simulink model "CyclingProcess_v2"  (R2022a)
settings: Solver=VariableStepAuto  StartTime=0.0  StopTime=10.0  RelTol=1e-3
settings Model: Creator=mateu  LastModifiedBy=mateu

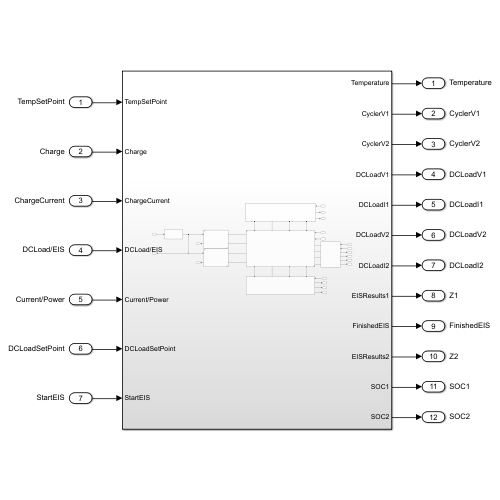
[thumbnail: Simulink's stored preview of the top-level diagram]
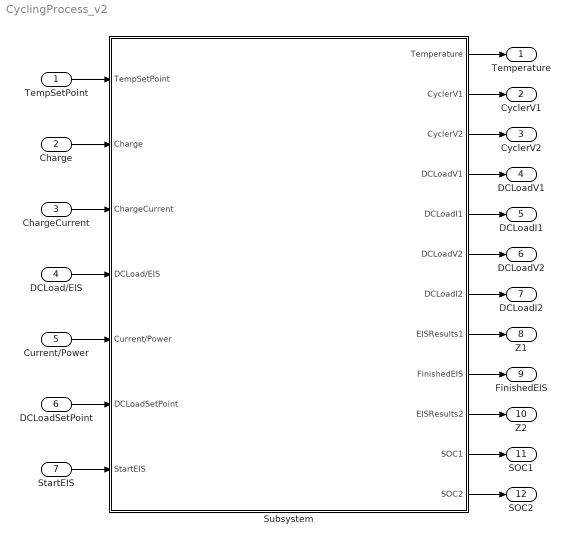
== system CyclingProcess_v2 ==
  TempSetPoint : Inport
  Charge : Inport  Port=2
  ChargeCurrent : Inport  Port=3
  DCLoad/EIS : Inport  Port=4
  Current/Power : Inport  Port=5
  DCLoadSetPoint : Inport  Port=6
  StartEIS : Inport  Port=7
  Subsystem : Subsystem
  Temperature : Outport
  CyclerV1 : Outport  Port=2
  CyclerV2 : Outport  Port=3
  DCLoadV1 : Outport  Port=4
  DCLoadI1 : Outport  Port=5
  DCLoadV2 : Outport  Port=6
  DCLoadI2 : Outport  Port=7
  Z1 : Outport  Port=8
  FinishedEIS : Outport  Port=9
  Z2 : Outport  Port=10
  SOC1 : Outport  Port=11
  SOC2 : Outport  Port=12
  wires:
  Subsystem/4(DCLoadV1) -> DCLoadV1/1
  Subsystem/7(DCLoadI2) -> DCLoadI2/1
  Subsystem/10(EISResults2) -> Z2/1
  Subsystem/12(SOC2) -> SOC2/1
  Subsystem/5(DCLoadI1) -> DCLoadI1/1
  Subsystem/11(SOC1) -> SOC1/1
  ChargeCurrent/1 -> Subsystem/3(ChargeCurrent)
  DCLoadSetPoint/1 -> Subsystem/6(DCLoadSetPoint)
  Subsystem/8(EISResults1) -> Z1/1
  Subsystem/3(CyclerV2) -> CyclerV2/1
  Charge/1 -> Subsystem/2(Charge)
  Subsystem/6(DCLoadV2) -> DCLoadV2/1
  Subsystem/1(Temperature) -> Temperature/1
  DCLoad/EIS/1 -> Subsystem/4(DCLoad/EIS)
  Current/Power/1 -> Subsystem/5(Current/Power)
  StartEIS/1 -> Subsystem/7(StartEIS)
  Subsystem/2(CyclerV1) -> CyclerV1/1
  TempSetPoint/1 -> Subsystem/1(TempSetPoint)
  Subsystem/9(FinishedEIS) -> FinishedEIS/1

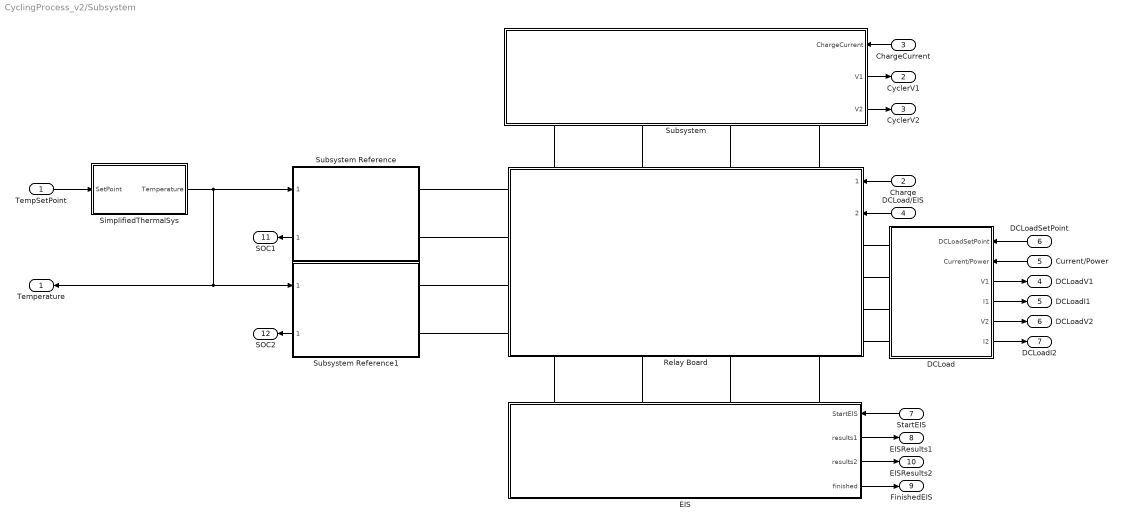
== system CyclingProcess_v2/Subsystem ==
  TempSetPoint : Inport
  Charge : Inport  Port=2
  ChargeCurrent : Inport  Port=3
  DCLoad/EIS : Inport  Port=4
  Current/Power : Inport  Port=5
  DCLoadSetPoint : Inport  Port=6
  StartEIS : Inport  Port=7
  DCLoad : Subsystem
      settings: PortSchema="{\"entries\":[{\"content\":{\"sides\":[{\"content\":{\"connectorIds\":[\"LConn1\",\"LConn2\",\"LConn3\",\"LConn4\"]},\"type\":\"ConnectorPlacement.EquallySpacedRectSide\",\"uuid\":\"7514b71b-63b4-4d0a-a4c6-1cc6fdc01e8b\"},{\"content\":{\"connectorIds\":[\"In1\",\"In2\",\"Out1\",\"Out2\",\"Out3\",\"Out4\"],\"side\":\"RIGHT\"},\"type\":\"ConnectorPlacement.EquallySpacedRectSide\",\"uuid\":\"8544a5e6-47c4-463c-a4b2-15ea7677f310\"},{\"content\":{\"connectorIds\":[],\"side\":\"TOP\"},\"type\":\"ConnectorPlacement.EquallySpacedRectSide\",\"uuid\":\"86aec749-4b5f-4df7-a96f-f425e3ea56a9\"}]},\"type\":\"ConnectorPlacement.EquallySpacedConnector\",\"uuid\":\"c9562699-1537-4762-a4d5-f653b7c21ddf\"}],\"packageUris\":[\"http://schema.mathworks.com/mf0/Connector/R2020b\"],\"version\":\"1.0\"}"
  EIS : Subsystem
      settings: PortSchema="{\"entries\":[{\"content\":{\"sides\":[{\"content\":{\"connectorIds\":[]},\"type\":\"ConnectorPlacement.EquallySpacedRectSide\",\"uuid\":\"cb9ec944-41ce-4636-a083-755c91ef9aeb\"},{\"content\":{\"connectorIds\":[\"In1\",\"Out1\",\"Out2\",\"Out3\"],\"side\":\"RIGHT\"},\"type\":\"ConnectorPlacement.EquallySpacedRectSide\",\"uuid\":\"d9055541-2ed5-47ee-9ebd-2502587374ee\"},{\"content\":{\"connectorIds\":[\"LConn1\",\"LConn2\",\"LConn3\",\"LConn4\"],\"side\":\"TOP\"},\"type\":\"ConnectorPlacement.EquallySpacedRectSide\",\"uuid\":\"957a55fb-9ef3-46c7-a91b-518a4a9602f1\"}]},\"type\":\"ConnectorPlacement.EquallySpacedConnector\",\"uuid\":\"9e8eff76-14a9-4e2b-897b-c7d74cf84e88\"}],\"packageUris\":[\"http://schema.mathworks.com/mf0/Connector/R2020b\"],\"version\":\"1.0\"}"
  Relay Board : Subsystem  ReferencedSubsystem=Relay_Board
      settings: PortSchema="{\"entries\":[{\"content\":{\"sides\":[{\"content\":{\"connectorIds\":[\"LConn1\",\"LConn2\",\"LConn3\",\"LConn4\"]},\"type\":\"ConnectorPlacement.EquallySpacedRectSide\",\"uuid\":\"b8d313c3-c08d-4f66-88c5-0966ca8ce19e\"},{\"content\":{\"connectorIds\":[\"In1\",\"In2\",\"RConn1\",\"RConn2\",\"RConn3\",\"RConn4\"],\"side\":\"RIGHT\"},\"type\":\"ConnectorPlacement.EquallySpacedRectSide\",\"uuid\":\"237515a3-1e1f-4c58-9863-54ac3610b1e3\"},{\"content\":{\"connectorIds\":[\"LConn5\",\"LConn6\",\"LConn7\",\"LConn8\"],\"side\":\"TOP\"},\"type\":\"ConnectorPlacement.EquallySpacedRectSide\",\"uuid\":\"521668e9-2c4f-424f-87c7-f56953ec1b76\"},{\"content\":{\"connectorIds\":[\"RConn5\",\"RConn6\",\"RConn7\",\"RConn8\"],\"side\":\"BOTTOM\"},\"type\":\"ConnectorPlacement.EquallySpacedRectSide\",\"uuid\":\"bf1ce9d0-6653-4dc3-bc27-a201294e6e6d\"}]},\"type\":\"ConnectorPlacement.EquallySpacedConnector\",\"uuid\":\"9b9e57dc-ee03-4c6e-905d-a66b18228b1b\"}],\"packageUris\":[\"http://schema.mathworks.com/mf0/Connector/R2020b\"],\"version\":\"1.0\"}"
  SimplifiedThermalSys : Subsystem
  Subsystem : Subsystem
      settings: PortSchema="{\"entries\":[{\"content\":{\"sides\":[{\"content\":{\"connectorIds\":[]},\"type\":\"ConnectorPlacement.EquallySpacedRectSide\",\"uuid\":\"cb9ec944-41ce-4636-a083-755c91ef9aeb\"},{\"content\":{\"connectorIds\":[\"In1\",\"Out1\",\"Out2\"],\"side\":\"RIGHT\"},\"type\":\"ConnectorPlacement.EquallySpacedRectSide\",\"uuid\":\"d9055541-2ed5-47ee-9ebd-2502587374ee\"},{\"content\":{\"connectorIds\":[],\"side\":\"TOP\"},\"type\":\"ConnectorPlacement.EquallySpacedRectSide\",\"uuid\":\"957a55fb-9ef3-46c7-a91b-518a4a9602f1\"},{\"content\":{\"connectorIds\":[\"RConn1\",\"RConn2\",\"RConn3\",\"RConn4\"],\"side\":\"BOTTOM\"},\"type\":\"ConnectorPlacement.EquallySpacedRectSide\",\"uuid\":\"144f5416-dcfd-4dc1-81f1-ec8b48bee9a2\"}]},\"type\":\"ConnectorPlacement.EquallySpacedConnector\",\"uuid\":\"9e8eff76-14a9-4e2b-897b-c7d74cf84e88\"}],\"packageUris\":[\"http://schema.mathworks.com/mf0/Connector/R2020b\"],\"version\":\"1.0\"}"
  Subsystem Reference : Subsystem  ReferencedSubsystem=Battery
      settings: PortSchema="{\"entries\":[{\"content\":{\"sides\":[{\"content\":{\"connectorIds\":[\"In1\",\"Out1\"]},\"type\":\"ConnectorPlacement.EquallySpacedRectSide\",\"uuid\":\"fc03161e-b2e2-4ac7-873d-06369879f611\"},{\"content\":{\"connectorIds\":[\"LConn1\",\"LConn2\"],\"side\":\"RIGHT\"},\"type\":\"ConnectorPlacement.EquallySpacedRectSide\",\"uuid\":\"979b6df9-5e16-4e4c-95de-06d721c40976\"},{\"content\":{\"connectorIds\":[],\"side\":\"TOP\"},\"type\":\"ConnectorPlacement.EquallySpacedRectSide\",\"uuid\":\"144c0b06-ab1a-42a6-a8bb-d1b96a840cfc\"}]},\"type\":\"ConnectorPlacement.EquallySpacedConnector\",\"uuid\":\"6783069b-24d2-410c-99c7-607924147892\"}],\"packageUris\":[\"http://schema.mathworks.com/mf0/Connector/R2020b\"],\"version\":\"1.0\"}"
  Subsystem Reference1 : Subsystem  ReferencedSubsystem=Battery
      settings: PortSchema="{\"entries\":[{\"content\":{\"sides\":[{\"content\":{\"connectorIds\":[\"In1\",\"Out1\"]},\"type\":\"ConnectorPlacement.EquallySpacedRectSide\",\"uuid\":\"fc03161e-b2e2-4ac7-873d-06369879f611\"},{\"content\":{\"connectorIds\":[\"LConn1\",\"LConn2\"],\"side\":\"RIGHT\"},\"type\":\"ConnectorPlacement.EquallySpacedRectSide\",\"uuid\":\"979b6df9-5e16-4e4c-95de-06d721c40976\"},{\"content\":{\"connectorIds\":[],\"side\":\"TOP\"},\"type\":\"ConnectorPlacement.EquallySpacedRectSide\",\"uuid\":\"144c0b06-ab1a-42a6-a8bb-d1b96a840cfc\"}]},\"type\":\"ConnectorPlacement.EquallySpacedConnector\",\"uuid\":\"6783069b-24d2-410c-99c7-607924147892\"}],\"packageUris\":[\"http://schema.mathworks.com/mf0/Connector/R2020b\"],\"version\":\"1.0\"}"
  Temperature : Outport
  CyclerV1 : Outport  Port=2
  CyclerV2 : Outport  Port=3
  DCLoadV1 : Outport  Port=4
  DCLoadI1 : Outport  Port=5
  DCLoadV2 : Outport  Port=6
  DCLoadI2 : Outport  Port=7
  EISResults1 : Outport  Port=8
  FinishedEIS : Outport  Port=9
  EISResults2 : Outport  Port=10
  SOC1 : Outport  Port=11
  SOC2 : Outport  Port=12
  wires:
  Subsystem Reference1/1 -> SOC2/1
  Subsystem Reference/1 -> SOC1/1
  Charge/1 -> Relay Board/1
  DCLoad/EIS/1 -> Relay Board/2
  SimplifiedThermalSys/1(Temperature) -> Subsystem Reference/1, Temperature/1, Subsystem Reference1/1
  TempSetPoint/1 -> SimplifiedThermalSys/1(SetPoint)
  DCLoadSetPoint/1 -> DCLoad/1(DCLoadSetPoint)
  Current/Power/1 -> DCLoad/2(Current/Power)
  DCLoad/1(V1) -> DCLoadV1/1
  DCLoad/2(I1) -> DCLoadI1/1
  DCLoad/3(V2) -> DCLoadV2/1
  DCLoad/4(I2) -> DCLoadI2/1
  EIS/2(results2) -> EISResults2/1
  EIS/1(results1) -> EISResults1/1
  StartEIS/1 -> EIS/1(StartEIS)
  Subsystem/2(V2) -> CyclerV2/1
  ChargeCurrent/1 -> Subsystem/1(ChargeCurrent)
  Subsystem/1(V1) -> CyclerV1/1
  EIS/3(finished) -> FinishedEIS/1
  connections:
  DCLoad/LConn4 -- Relay Board/RConn4
  DCLoad/LConn3 -- Relay Board/RConn3
  Subsystem Reference/LConn1 -- Relay Board/LConn1
  Subsystem Reference/LConn2 -- Relay Board/LConn2
  Relay Board/RConn2 -- DCLoad/LConn2
  Subsystem Reference1/LConn1 -- Relay Board/LConn3
  Subsystem Reference1/LConn2 -- Relay Board/LConn4
  Relay Board/RConn1 -- DCLoad/LConn1
  EIS/LConn1 -- Relay Board/RConn5
  EIS/LConn2 -- Relay Board/RConn6
  EIS/LConn3 -- Relay Board/RConn7
  EIS/LConn4 -- Relay Board/RConn8
  Subsystem/RConn1 -- Relay Board/LConn5
  Subsystem/RConn2 -- Relay Board/LConn6
  Subsystem/RConn3 -- Relay Board/LConn7
  Subsystem/RConn4 -- Relay Board/LConn8

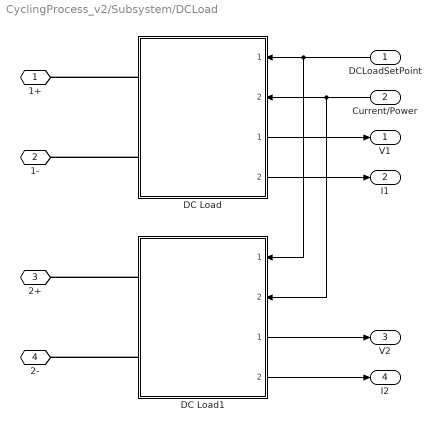
== system CyclingProcess_v2/Subsystem/DCLoad ==
  DCLoadSetPoint : Inport
  Current/Power : Inport  Port=2
  DC Load : Subsystem  ReferencedSubsystem=DC_Load
      settings: PortSchema="{\"entries\":[{\"content\":{\"sides\":[{\"content\":{\"connectorIds\":[\"LConn1\",\"LConn2\"]},\"type\":\"ConnectorPlacement.EquallySpacedRectSide\",\"uuid\":\"747fffec-1188-4560-a63f-e796ff73abc9\"},{\"content\":{\"connectorIds\":[\"In1\",\"In2\",\"Out1\",\"Out2\"],\"side\":\"RIGHT\"},\"type\":\"ConnectorPlacement.EquallySpacedRectSide\",\"uuid\":\"c8b2c27b-57f0-426f-8f7f-d4e2bbdef76e\"},{\"content\":{\"connectorIds\":[],\"side\":\"TOP\"},\"type\":\"ConnectorPlacement.EquallySpacedRectSide\",\"uuid\":\"aa3beff7-3052-4685-a7af-7f3c81e4b1e5\"}]},\"type\":\"ConnectorPlacement.EquallySpacedConnector\",\"uuid\":\"a83fffc3-2d86-4bd9-832d-7e01edf78d97\"}],\"packageUris\":[\"http://schema.mathworks.com/mf0/Connector/R2020b\"],\"version\":\"1.0\"}"
  DC Load1 : Subsystem  ReferencedSubsystem=DC_Load
      settings: PortSchema="{\"entries\":[{\"content\":{\"sides\":[{\"content\":{\"connectorIds\":[\"LConn1\",\"LConn2\"]},\"type\":\"ConnectorPlacement.EquallySpacedRectSide\",\"uuid\":\"747fffec-1188-4560-a63f-e796ff73abc9\"},{\"content\":{\"connectorIds\":[\"In1\",\"In2\",\"Out1\",\"Out2\"],\"side\":\"RIGHT\"},\"type\":\"ConnectorPlacement.EquallySpacedRectSide\",\"uuid\":\"c8b2c27b-57f0-426f-8f7f-d4e2bbdef76e\"},{\"content\":{\"connectorIds\":[],\"side\":\"TOP\"},\"type\":\"ConnectorPlacement.EquallySpacedRectSide\",\"uuid\":\"aa3beff7-3052-4685-a7af-7f3c81e4b1e5\"}]},\"type\":\"ConnectorPlacement.EquallySpacedConnector\",\"uuid\":\"a83fffc3-2d86-4bd9-832d-7e01edf78d97\"}],\"packageUris\":[\"http://schema.mathworks.com/mf0/Connector/R2020b\"],\"version\":\"1.0\"}"
  1+ : PMIOPort  Side=Left
  1- : PMIOPort  Port=2  Side=Left
  2+ : PMIOPort  Port=3  Side=Left
  2- : PMIOPort  Port=4  Side=Left
  V1 : Outport
  I1 : Outport  Port=2
  V2 : Outport  Port=3
  I2 : Outport  Port=4
  wires:
  DCLoadSetPoint/1 -> DC Load1/1, DC Load/1
  Current/Power/1 -> DC Load1/2, DC Load/2
  DC Load/1 -> V1/1
  DC Load/2 -> I1/1
  DC Load1/1 -> V2/1
  DC Load1/2 -> I2/1
  connections:
  DC Load/LConn1 -- 1+/RConn1
  DC Load/LConn2 -- 1-/RConn1
  DC Load1/LConn1 -- 2+/RConn1
  DC Load1/LConn2 -- 2-/RConn1

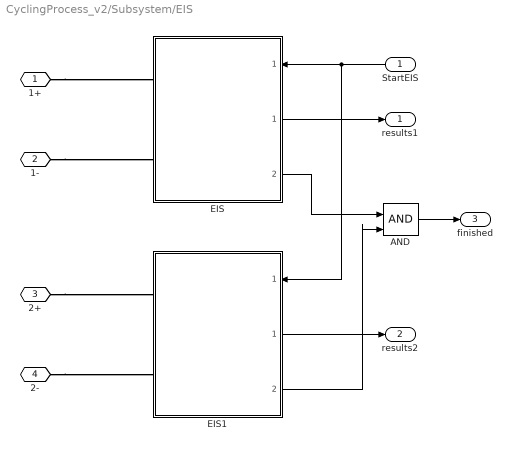
== system CyclingProcess_v2/Subsystem/EIS ==
  StartEIS : Inport
  AND : Logic  IconShape=distinctive  AllPortsSameDT=off  OutDataTypeStr=boolean
  EIS : Subsystem  ReferencedSubsystem=EIS
      settings: PortSchema="{\"entries\":[{\"content\":{\"sides\":[{\"content\":{\"connectorIds\":[\"LConn1\",\"LConn2\"]},\"type\":\"ConnectorPlacement.EquallySpacedRectSide\",\"uuid\":\"b4295795-bb4f-4226-ae08-13ff31e69c7e\"},{\"content\":{\"connectorIds\":[\"In1\",\"Out1\",\"Out2\"],\"side\":\"RIGHT\"},\"type\":\"ConnectorPlacement.EquallySpacedRectSide\",\"uuid\":\"cf500fd2-35e2-47f1-8094-2f89cbc86857\"},{\"content\":{\"connectorIds\":[],\"side\":\"TOP\"},\"type\":\"ConnectorPlacement.EquallySpacedRectSide\",\"uuid\":\"635a65a1-d415-436a-9540-513bae37053e\"}]},\"type\":\"ConnectorPlacement.EquallySpacedConnector\",\"uuid\":\"170704b4-cdd6-4628-9347-edd0fb851791\"}],\"packageUris\":[\"http://schema.mathworks.com/mf0/Connector/R2020b\"],\"version\":\"1.0\"}"
  EIS1 : Subsystem  ReferencedSubsystem=EIS
      settings: PortSchema="{\"entries\":[{\"content\":{\"sides\":[{\"content\":{\"connectorIds\":[\"LConn1\",\"LConn2\"]},\"type\":\"ConnectorPlacement.EquallySpacedRectSide\",\"uuid\":\"b4295795-bb4f-4226-ae08-13ff31e69c7e\"},{\"content\":{\"connectorIds\":[\"In1\",\"Out1\",\"Out2\"],\"side\":\"RIGHT\"},\"type\":\"ConnectorPlacement.EquallySpacedRectSide\",\"uuid\":\"cf500fd2-35e2-47f1-8094-2f89cbc86857\"},{\"content\":{\"connectorIds\":[],\"side\":\"TOP\"},\"type\":\"ConnectorPlacement.EquallySpacedRectSide\",\"uuid\":\"635a65a1-d415-436a-9540-513bae37053e\"}]},\"type\":\"ConnectorPlacement.EquallySpacedConnector\",\"uuid\":\"170704b4-cdd6-4628-9347-edd0fb851791\"}],\"packageUris\":[\"http://schema.mathworks.com/mf0/Connector/R2020b\"],\"version\":\"1.0\"}"
  1+ : PMIOPort  Side=Left
  1- : PMIOPort  Port=2  Side=Left
  2+ : PMIOPort  Port=3  Side=Left
  2- : PMIOPort  Port=4  Side=Left
  results1 : Outport
  results2 : Outport  Port=2
  finished : Outport  Port=3
  wires:
  StartEIS/1 -> EIS1/1, EIS/1
  EIS/1 -> results1/1
  EIS1/1 -> results2/1
  EIS/2 -> AND/1
  EIS1/2 -> AND/2
  AND/1 -> finished/1
  connections:
  1+/RConn1 -- EIS/LConn1
  1-/RConn1 -- EIS/LConn2
  2+/RConn1 -- EIS1/LConn1
  2-/RConn1 -- EIS1/LConn2

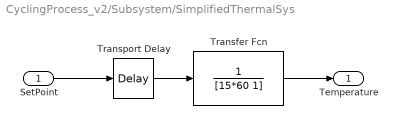
== system CyclingProcess_v2/Subsystem/SimplifiedThermalSys ==
  SetPoint : Inport
  Transfer Fcn : TransferFcn  Denominator=[15*60 1]
  Transport Delay : TransportDelay  DelayTime=5
  Temperature : Outport
  wires:
  Transport Delay/1 -> Transfer Fcn/1
  SetPoint/1 -> Transport Delay/1
  Transfer Fcn/1 -> Temperature/1

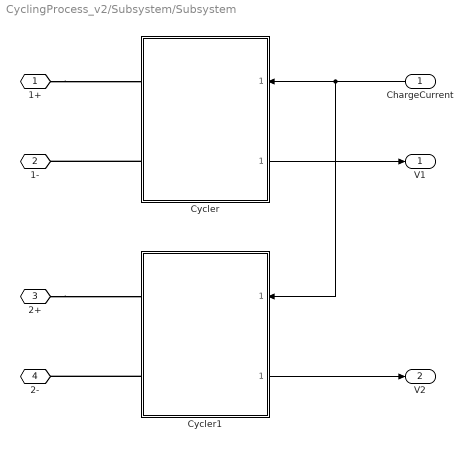
== system CyclingProcess_v2/Subsystem/Subsystem ==
  ChargeCurrent : Inport
  Cycler : Subsystem  ReferencedSubsystem=Cycler
      settings: PortSchema="{\"entries\":[{\"content\":{\"sides\":[{\"content\":{\"connectorIds\":[\"RConn1\",\"RConn2\"]},\"type\":\"ConnectorPlacement.EquallySpacedRectSide\",\"uuid\":\"ea079f9a-06f7-44f0-82a3-29caf877d5c1\"},{\"content\":{\"connectorIds\":[\"In1\",\"Out1\"],\"side\":\"RIGHT\"},\"type\":\"ConnectorPlacement.EquallySpacedRectSide\",\"uuid\":\"2059dbe0-ef1b-4ded-af29-4eaf93ad6300\"},{\"content\":{\"connectorIds\":[],\"side\":\"TOP\"},\"type\":\"ConnectorPlacement.EquallySpacedRectSide\",\"uuid\":\"8df91527-c275-4289-bf22-8cb26e616748\"},{\"content\":{\"connectorIds\":[],\"side\":\"BOTTOM\"},\"type\":\"ConnectorPlacement.EquallySpacedRectSide\",\"uuid\":\"caed2e17-fe93-476b-b416-bef95d6befc0\"}]},\"type\":\"ConnectorPlacement.EquallySpacedConnector\",\"uuid\":\"3ec12977-8066-4dcd-bce9-b6d1ce2c81ea\"}],\"packageUris\":[\"http://schema.mathworks.com/mf0/Connector/R2020b\"],\"version\":\"1.0\"}"
  Cycler1 : Subsystem  ReferencedSubsystem=Cycler
      settings: PortSchema="{\"entries\":[{\"content\":{\"sides\":[{\"content\":{\"connectorIds\":[\"RConn1\",\"RConn2\"]},\"type\":\"ConnectorPlacement.EquallySpacedRectSide\",\"uuid\":\"ea079f9a-06f7-44f0-82a3-29caf877d5c1\"},{\"content\":{\"connectorIds\":[\"In1\",\"Out1\"],\"side\":\"RIGHT\"},\"type\":\"ConnectorPlacement.EquallySpacedRectSide\",\"uuid\":\"2059dbe0-ef1b-4ded-af29-4eaf93ad6300\"},{\"content\":{\"connectorIds\":[],\"side\":\"TOP\"},\"type\":\"ConnectorPlacement.EquallySpacedRectSide\",\"uuid\":\"8df91527-c275-4289-bf22-8cb26e616748\"},{\"content\":{\"connectorIds\":[],\"side\":\"BOTTOM\"},\"type\":\"ConnectorPlacement.EquallySpacedRectSide\",\"uuid\":\"caed2e17-fe93-476b-b416-bef95d6befc0\"}]},\"type\":\"ConnectorPlacement.EquallySpacedConnector\",\"uuid\":\"3ec12977-8066-4dcd-bce9-b6d1ce2c81ea\"}],\"packageUris\":[\"http://schema.mathworks.com/mf0/Connector/R2020b\"],\"version\":\"1.0\"}"
  1+ : PMIOPort  Side=Right
  1- : PMIOPort  Port=2  Side=Right
  2+ : PMIOPort  Port=3  Side=Right
  2- : PMIOPort  Port=4  Side=Right
  V1 : Outport
  V2 : Outport  Port=2
  wires:
  ChargeCurrent/1 -> Cycler1/1, Cycler/1
  Cycler/1 -> V1/1
  Cycler1/1 -> V2/1
  connections:
  1+/RConn1 -- Cycler/RConn1
  2+/RConn1 -- Cycler1/RConn1
  Cycler1/RConn2 -- 2-/RConn1
  Cycler/RConn2 -- 1-/RConn1
